simulink model "fuelcell_adapt_cs"  (Simulink 4.00)
settings: Solver=ode1  SolverMode=SingleTasking  StartTime=0.0  StopTime=29  FixedStep=1  RelTol=1e-3
undefined symbols (not defined in the file or in its folder): EssAdaptTime, FcReqAdaptPwr
libraries: lib_fuel_cell x1
settings Model: LastModifiedBy=bjeanner  AlgebraicLoopMsg=none  UnconnectedInputMsg=none  UnconnectedOutputMsg=none  UnconnectedLineMsg=none  InheritedTsInSrcMsg=none  IntegerOverflowMsg=none  Int32ToFloatConvMsg=none

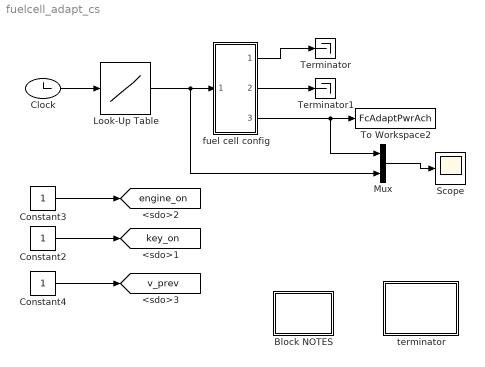
== system fuelcell_adapt_cs ==
  Block NOTES : Subsystem
      settings: RTWFcnNameOpts=Auto  RTWFileNameOpts=Auto
      mask Display: disp('Block\nNOTES')
  Clock : Clock
  Constant2 : Constant  Value=1
  Constant3 : Constant  Value=1
  Constant4 : Constant  Value=1
  Look-Up Table : Lookup  InputValues=EssAdaptTime  OutputValues=FcReqAdaptPwr
  Mux : Mux  Inputs=2
  Scope : Scope
      settings: TimeRange=auto  YMin=-5  YMax=5  SaveToWorkspace=off  SaveName=ScopeData  LimitDataPoints=on  MaxDataPoints=5000
  Terminator : Terminator
  Terminator1 : Terminator
  To Workspace2 : ToWorkspace  VariableName=FcAdaptPwrAch  SampleTime=-1  SaveFormat=Array
  fuel cell config : Subsystem  BlockChoice=fuel converter <fc> VT model
      settings: AttributesFormatString=%<BlockChoice>  TemplateBlock=lib_fuel_cell/fuel cell config  MemberBlocks="fuel converter <fc>  KTH fc model,fuel converter <fc> GCTool linkage,fuel converter <fc> VT model,fuel converter <fc> net model,fuel converter <fc> polarization curve model"  RTWFcnNameOpts=Auto  RTWFileNameOpts=Auto
  terminator : Subsystem
      settings: RTWFcnNameOpts=Auto  RTWFileNameOpts=Auto
  tag scope: engine_on=global, key_on=global, v_prev=global
  wires:
  Look-Up Table/1 -> fuel cell config/1(pwr req'd at fc  output (W)), Mux/2
  fuel cell config/1(fuel use) -> Terminator/1
  fuel cell config/2(EO emis info) -> Terminator1/1
  fuel cell config/3(pwr avail. to driveline (W)) -> To Workspace2/1, Mux/1
  Constant2/1 -> [key_on]
  Constant3/1 -> [engine_on]
  Constant4/1 -> [v_prev]
  Clock/1 -> Look-Up Table/1
  Mux/1 -> Scope/1

== system fuelcell_adapt_cs/Block NOTES ==
  note: This block diagram runs with the fuel cell adaptive control strategy.
      | It is called by the sfun_fuelcell_adapt.m script.
      |
      | Input:
      | Power required from the fuel cell (assign in the sfunction)
      | Output:
      | Mass flow fuel consumption: fc_fuel_rate

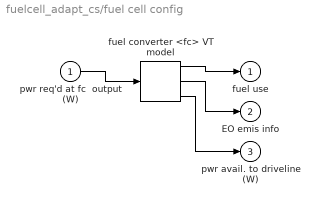
== system fuelcell_adapt_cs/fuel cell config ==
  pwr req'd at fc  output (W) : Inport  Port=1  LatchInput=off
  fuel converter <fc> VT model : lib_fuel_cell/fuel converter <fc> VT model
  fuel use : Outport  Port=1
  EO emis info : Outport  Port=2
  pwr avail. to driveline (W) : Outport  Port=3
  wires:
  pwr req'd at fc  output (W)/1 -> fuel converter <fc> VT model/1
  fuel converter <fc> VT model/1 -> fuel use/1
  fuel converter <fc> VT model/2 -> EO emis info/1
  fuel converter <fc> VT model/3 -> pwr avail. to driveline (W)/1

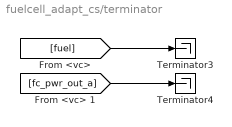
== system fuelcell_adapt_cs/terminator ==
  Terminator3 : Terminator
  Terminator4 : Terminator
  wires:
  [fuel] -> Terminator3/1
  [fc_pwr_out_a] -> Terminator4/1
